simulink model "VTOL_quadplane"  (R2026a)
settings: Solver=ode1  StopTime=120  FixedStep=1/60  MaxStep=0.01
undefined symbols (not defined in the file or in its folder): op_trim, params, Receive, Send
libraries: slpidlib x32, simulink_extras x11, simulink x2, aerolibfltsims x2, aerolibobsolete x1, sim3dlib x1, uavsim3dlib x1
(part 1 of 4)
settings Model: Creator=Admin  LastModifiedBy=Admin
settings DebuggingCC: InheritedTsInSrcMsg=none

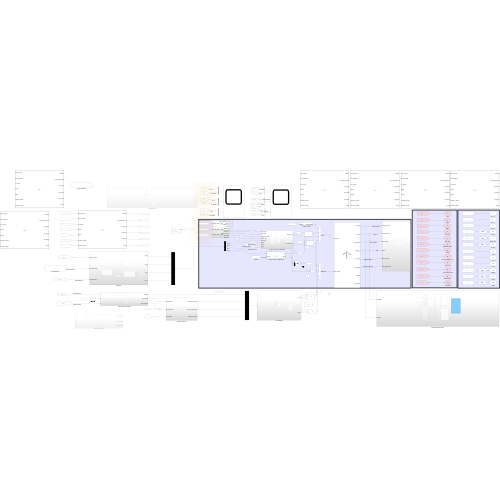
[thumbnail: Simulink's stored preview of the top-level diagram]
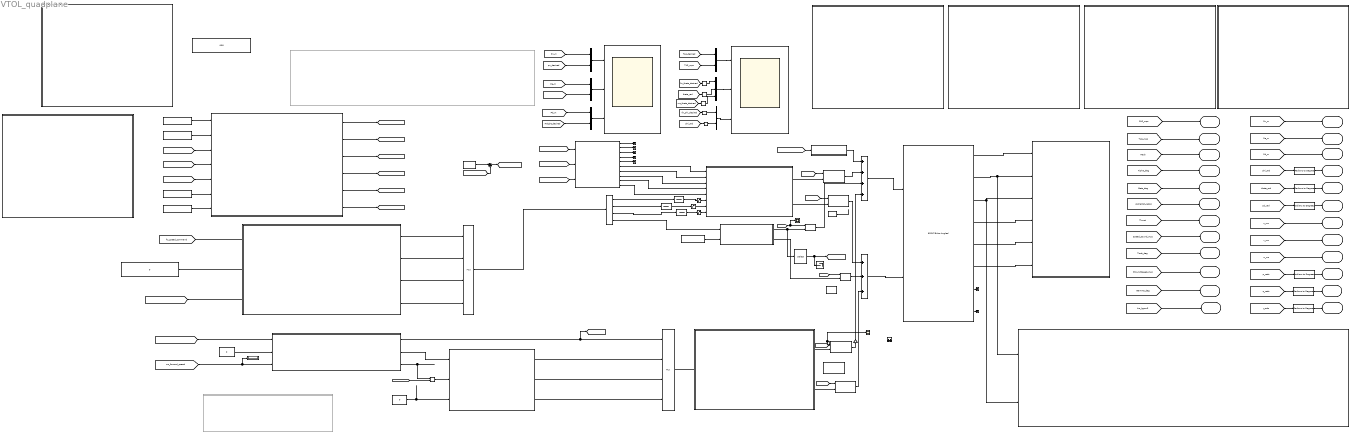
== system VTOL_quadplane ==
  note: Fixed Wing Dynamics
  6DOF (Euler Angles) : aerolibobsolete/6DOF (Euler Angles)  units=Metric (MKS)  mtype=Fixed  rep=Euler Angles  xme_0=[0;0;-1]  Vm_0=[0.01;0;0]  eul_0=[0;0;0]  pm_0=[0;0;0]  mass_0=params.geometric.mass  mass_e=0.5  mass_f=2.0  inertia=params.geometric.I  inertia_e=eye(3)  inertia_f=2*eye(3)  k_quat=1.0  vre_flag=on  abi_flag=off  aMode=0  xme_statename=''  Vm_statename=''  eul_statename=''  quat_statename=''  pm_statename=''  mass_statename=''
  Actuator_servo 1 : TransferFcn  Denominator=[0.02 1]
  Actuator_servo 2 : TransferFcn  Denominator=[0.02 1]
  Actuator_servo 3 : TransferFcn  Denominator=[0.02 1]
  Add : Sum  Inputs=++++
  Add1 : Sum  Inputs=+++
  Add3 : Sum
  Aero_Forces_and_Moments : Subsystem
  Attitude Controller : Subsystem
  Autopilot : Subsystem
  Constant : Constant  Value=24
  Constant1 : Constant  Value=0
  Constant2 : Constant  Value=0
  Constant3 : Constant  Value=-75
  Constant4 : Constant  Value=18
  Constant5 : Constant  Value=0
  Constant7 : Constant
  Constant9 : Constant  Value=-50
  Course Desired : Constant  Value=0
  Course Desired1 : Constant  Value=-100
  Demux : Demux
  Display1 : Display
  Gain : Gain
  Gravity_forces : Subsystem
  MATLAB Function1 : MATLAB Function  TreatAsAtomicUnit=on
  MATLAB Function2 : MATLAB Function  TreatAsAtomicUnit=on
  MATLAB Function3 : MATLAB Function  TreatAsAtomicUnit=on
  MATLAB Function4 : MATLAB Function  TreatAsAtomicUnit=on
  MATLAB Function5 : MATLAB Function  TreatAsAtomicUnit=on
  MATLAB Function6 : MATLAB Function  TreatAsAtomicUnit=on
  MATLAB Function7 : MATLAB Function  TreatAsAtomicUnit=on
  Motor Mixing : Subsystem
  Mux{,1,4,6..7} (5 alike) : Mux  Inputs=2
  Mux2 : Mux
  Mux5 : Mux  Inputs=3
  Mux8 : Mux
  Position Controller1 : Subsystem  Commented=on
  Product{,1..5,8..10} (9 alike) : Product
  Pusher Forces and Moments : MATLAB Function  TreatAsAtomicUnit=on
  Quad Velocity Controller : Subsystem
  Radians to Degrees{,1..4,11..16} (11 alike) : simulink_extras/Transformations/Radians to Degrees
  Saturation1 : Saturate  UpperLimit=deg2rad(25)  LowerLimit=deg2rad(-25)
  Saturation2 : Saturate  UpperLimit=deg2rad(25)  LowerLimit=deg2rad(-25)
  Saturation4 : Saturate  UpperLimit=deg2rad(25)  LowerLimit=deg2rad(-25)
  Scope : Scope  NumInputPorts=3
      settings: ActiveDisplayYMinimum=-441.15296890971007  ActiveDisplayYMaximum=3970.3767201873916
  Scope1 : Scope  NumInputPorts=3
      settings: ActiveDisplayYMinimum=-3.1220021954441637  ActiveDisplayYMaximum=28.098019758997481
  Scope2 : Scope
      settings: ActiveDisplayYMinimum=-1  ActiveDisplayYMaximum=1  DataLoggingVariableName=ScopeData2
  Scope3 : Scope
      settings: ActiveDisplayYMinimum=-0.12499999999999997  ActiveDisplayYMaximum=1.125  DataLoggingVariableName=ScopeData3
  Selector : Selector  InputPortWidth=3  IndexOptions=Index vector (dialog)  Indices=[1]  OutputSizes=1
  Subsystem1 : Subsystem
  Subsystem2 : Subsystem
  Sum : Sum  Inputs=|+-
  Terminator{1..8} (8 alike) : Terminator
  Transition Block : Subsystem  Commented=on
  Visualisation Subsystem : Subsystem
  params1 : Constant  Value=params  OutDataTypeStr=Bus: slBus1
  CAS : Outport
  TAS : Outport  Port=2
  Mach : Outport  Port=3
  Alpha_deg : Outport  Port=4
  Beta_deg : Outport  Port=5
  AlphaDot_radps : Outport  Port=6
  Pn_m : Outport  Port=7
  Pe_m : Outport  Port=8
  Pd_m : Outport  Port=9
  Phi_deg : Outport  Port=10
  Theta_deg : Outport  Port=11
  Psi_deg : Outport  Port=12
  u_ms : Outport  Port=13
  v_ms : Outport  Port=14
  w_ms : Outport  Port=15
  p_deg/s : Outport  Port=16
  q_deg/s : Outport  Port=17
  r_deg/s : Outport  Port=18
  Thrust : Outport  Port=19
  Speed_Sound_mps : Outport  Port=20
  Track_deg : Outport  Port=21
  Ground Speed m/s : Outport  Port=22
  rho_kgpm3 : Outport  Port=23
  Gamma_deg : Outport  Port=24
  tag scope: Thrust=global, fw_height_command=global, fw_speed_command=global, lambda=global, mc_forward_speed=global, mc_height_command=global, mode=global, one_minus_lambda=global, throttle=global
  wires:
  [CAS_mps] -> CAS/1
  [TAS_mps] -> TAS/1
  [Mach] -> Mach/1
  [Alpha_deg] -> Alpha_deg/1
  [Beta_deg] -> Beta_deg/1
  [AlphaDot_radps] -> AlphaDot_radps/1
  [Pn_m] -> Pn_m/1
  [Pe_m] -> Pe_m/1
  [Pd_m] -> Pd_m/1
  [phi_rad] -> Radians to Degrees11/1
  Radians to Degrees11/1 -> Phi_deg/1
  Radians to Degrees12/1 -> Theta_deg/1
  [theta_rad] -> Radians to Degrees12/1
  Radians to Degrees13/1 -> Psi_deg/1
  [psi_rad] -> Radians to Degrees13/1
  [u_ms] -> u_ms/1
  [v_ms] -> v_ms/1
  [w_ms] -> w_ms/1
  [p_rads] -> Radians to Degrees14/1
  Radians to Degrees14/1 -> p_deg/s/1
  [q_rads] -> Radians to Degrees15/1
  Radians to Degrees15/1 -> q_deg/s/1
  [r_rads] -> Radians to Degrees16/1
  Radians to Degrees16/1 -> r_deg/s/1
  [Thrust] -> Thrust/1
  [Speed_Sound_mps] -> Speed_Sound_mps/1
  [Track_deg] -> Track_deg/1
  [GroundSpeed_mps] -> Ground Speed m/s/1
  [rho_kgpm3] -> rho_kgpm3/1
  [Gamma_deg] -> Gamma_deg/1
  ? -> ?
  Course Desired/1 -> Autopilot/2(Course Desired)  "Course Desired"
  Autopilot/1(Del_a) -> Mux8/1
  Autopilot/2(Del_e) -> Mux8/2
  Autopilot/3(Del_r) -> Mux8/3
  Autopilot/4(Del_T) -> Mux8/4
  Subsystem1/5(CAS_mps) -> Terminator5/1
  6DOF (Euler Angles)/3 -> Visualisation Subsystem/2(Rotation), Subsystem2/3(Euler angles)  "Euler angles"
  6DOF (Euler Angles)/1 -> Subsystem2/1(Inertial_Velocity)  "Inertial Velocity"
  [Inertial_Wind_Z] -> Subsystem1/3(Inertial_Wind_Z_mps)
  params1/1 -> Pusher Forces and Moments/2(params)
  Subsystem1/3(Pressure_Pa) -> Terminator3/1
  Subsystem1/4(Mach) -> Terminator4/1
  [Inertial_Wind_X] -> Subsystem1/1(Inertial_Wind_X_mps)
  Aero_Forces_and_Moments/2(Aero_Moments) -> Product3/2
  Subsystem1/9(Alpha_deg) -> Aero_Forces_and_Moments/4(Alpha_deg)
  Add1/1 -> 6DOF (Euler Angles)/2  "Moments"
  Subsystem1/2(Temp k) -> Terminator2/1
  6DOF (Euler Angles)/5 -> Subsystem2/5(Body Velocities)  "Body Velocities"
  6DOF (Euler Angles)/8 -> Terminator7/1
  Demux/1 -> Actuator_servo 1/1  "Del_a"
  Subsystem1/6(rho_kgpm3) -> Aero_Forces_and_Moments/1(rho_kgpm)
  Subsystem1/8(AlphaDot_radps) -> Aero_Forces_and_Moments/3(AlphaDot_radps)
  Subsystem1/1(Speed_Sound_mps) -> Terminator1/1
  6DOF (Euler Angles)/7 -> Terminator6/1
  Subsystem1/7(TAS_mps) -> Aero_Forces_and_Moments/2(TAS_mps)
  Add/1 -> 6DOF (Euler Angles)/1  "forces"
  [DCM] -> Gravity_forces/1(DCM)
  6DOF (Euler Angles)/4 -> Subsystem2/4(DCM)  "DCM"
  Subsystem1/10(Beta_deg) -> Aero_Forces_and_Moments/5(Beta_deg)
  Gravity_forces/1(Gravity_forces) -> Add/1
  [Inertial_Wind_Y] -> Subsystem1/2(Inertial_Wind_Y_mps)
  6DOF (Euler Angles)/2 -> Visualisation Subsystem/1(Translation), Subsystem2/2(Inertial_Position)  "Postion"
  Selector/1 -> [Thrust], Terminator8/1
  6DOF (Euler Angles)/6 -> Subsystem2/6(body angular rates)  "body angular rates"
  Mux8/1 -> Demux/1
  Quad Velocity Controller/1(Throttle) -> [throttle], Mux2/1
  Mux2/1 -> Motor Mixing/1(In1)
  Attitude Controller/1(Roll Control Torque) -> Mux2/2
  Attitude Controller/2(Pitch Control Torque) -> Mux2/3
  [mc_height_command] -> Quad Velocity Controller/1(In1)  "Height Desired"
  Attitude Controller/3(Yaw Control Torque) -> Mux2/4
  Constant2/1 -> Quad Velocity Controller/2(In2)
  Motor Mixing/1(F_vtol) -> Product1/2
  Motor Mixing/2(M_xyz) -> Product/2
  Constant5/1 -> Attitude Controller/3(Psi_desired)
  Product/1 -> Add1/3
  [Pd_m] -> Mux7/1  "Pd_m"
  [Pn_m] -> Mux1/1  "Pn_m"
  [pe_desired] -> Mux/2  "pe_desired"
  [Pe_m] -> Mux/1  "pe_m"
  Mux1/1 -> Scope/1
  [pn_desired] -> Mux1/2  "pn_desired"
  [Height_desired] -> Mux7/2  "Pd_desired"
  Mux/1 -> Scope/2
  Mux7/1 -> Scope/3
  [one_minus_lambda] -> Product/1
  [one_minus_lambda] -> Scope2/1, Product1/1
  Product1/1 -> Gain/1
  Aero_Forces_and_Moments/1(Aero_forces) -> Product2/2
  [lambda] -> Product2/1
  Product3/1 -> Add1/1
  [lambda] -> Product3/1
  Product2/1 -> Add/2
  Mux4/1 -> Scope1/1
  Mux5/1 -> Scope1/2
  Mux6/1 -> Scope1/3
  [Tas_desired] -> Mux4/1  "V-desired"
  [TAS_mps] -> Mux4/2  "Vms"
  [fw_theta_desired] -> Radians to Degrees/1
  [theta_rad] -> Radians to Degrees1/1
  [fw_phi_desired] -> Radians to Degrees2/1
  Radians to Degrees/1 -> Mux5/1  "Theta_desired"
  Radians to Degrees1/1 -> Mux5/2  "Theta"
  Radians to Degrees2/1 -> Mux6/1  "Phi_desired"
  [phi_rad] -> Radians to Degrees3/1
  Radians to Degrees3/1 -> Mux6/2  "Phi"
  Quad Velocity Controller/2(Phi_desired) -> Attitude Controller/1(Phi_desired)
  [fw_height_command] -> Autopilot/3(Height Desired)  "Height Desired"
  Constant1/1 -> ?
  Constant7/1 -> Sum/1
  Demux/4 -> Pusher Forces and Moments/1(u)  "Del_T"
  [lambda] -> Sum/2
  Sum/1 -> [one_minus_lambda]
  Actuator_servo 1/1 -> Saturation4/1
  Actuator_servo 2/1 -> Saturation1/1
  Actuator_servo 3/1 -> Saturation2/1
  [mc_forward_speed] -> Display1/1, Quad Velocity Controller/3(In3)  "Height Desired"
  [lambda] -> Product9/1, Scope3/1
  Pusher Forces and Moments/2(M_fw) -> Product5/2
  [lambda] -> Product5/1
  Quad Velocity Controller/3(Theta_desired) -> Product8/1
  Demux/3 -> Actuator_servo 3/1  "Del_r"
  Demux/2 -> Actuator_servo 2/1  "Del_e"
  [fw_speed_command] -> Autopilot/1(Speed_desired)  "Speed_desired"
  Pusher Forces and Moments/1(F_fw) -> Product9/2, Selector/1
  Product5/1 -> Add1/2
  Saturation4/1 -> Aero_Forces_and_Moments/6(Del_a)
  Saturation2/1 -> Aero_Forces_and_Moments/8(Del_r)
  Constant/1 -> MATLAB Function1/1(cruise_speed)
  MATLAB Function1/5(fw_height) -> [fw_height_command]
  Constant4/1 -> MATLAB Function1/6(transition_speed)
  MATLAB Function1/2(mc_forward_speed) -> [mc_forward_speed]
  Constant3/1 -> MATLAB Function1/2(cruise_altitude)
  MATLAB Function1/3(mc_height) -> [mc_height_command]
  MATLAB Function1/4(fw_speed) -> [fw_speed_command]
  [Pd_m] -> MATLAB Function1/5(height)
  Constant9/1 -> MATLAB Function1/7(transition_height)
  MATLAB Function1/6(mode) -> [mode]
  MATLAB Function1/1(lambda) -> [lambda]
  [TAS_mps] -> MATLAB Function1/3(mc_speed)
  [TAS_mps] -> MATLAB Function1/4(speed)
  [one_minus_lambda] -> Product8/2
  Product8/1 -> Attitude Controller/2(Theta_desired)
  Product9/1 -> Add/3
  Gain/1 -> Add/4
  Saturation1/1 -> Aero_Forces_and_Moments/7(Del_e)
  [mc_theta_desired] -> Radians to Degrees4/1
  Radians to Degrees4/1 -> Mux5/3  "mc_Theta_desired"

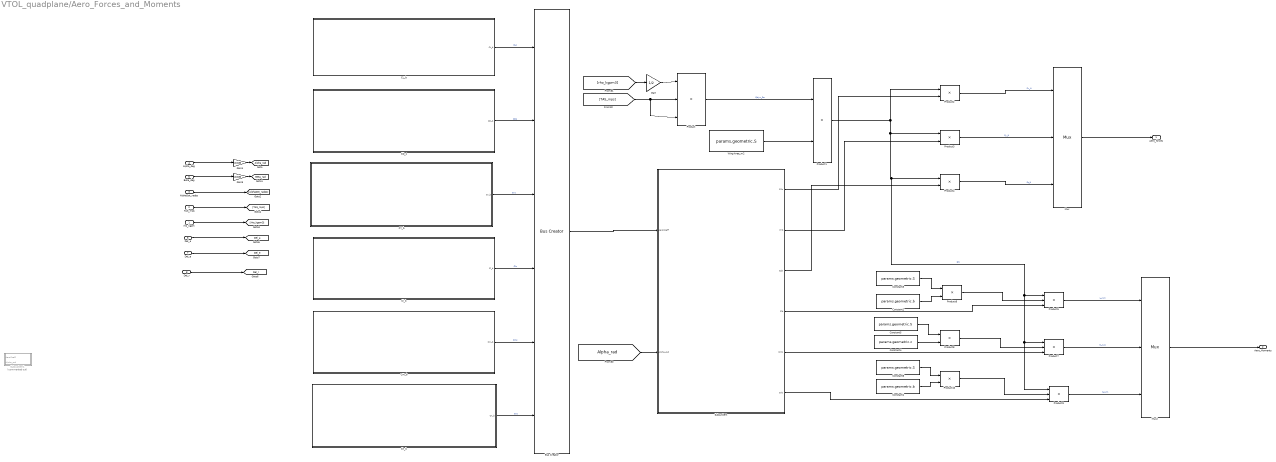
== system VTOL_quadplane/Aero_Forces_and_Moments ==
  rho_kgpm : Inport
  TAS_mps : Inport  Port=2
  AlphaDot_radps : Inport  Port=3
  Alpha_deg : Inport  Port=4
  Beta_deg : Inport  Port=5
  Del_a : Inport  Port=6
  Del_e : Inport  Port=7
  Del_r : Inport  Port=8
  Bus Creator : BusCreator  Inputs=6
  CD_s : Subsystem
  CL_b : Subsystem
  CY_b : Subsystem
  Cl_b : Subsystem
  Cm_b : Subsystem
  Cn_b : Subsystem
  Constant1 : Constant  Value=params.geometric.b
  Constant2 : Constant  Value=params.geometric.b
  Constant3 : Constant  Value=params.geometric.S
  Constant4 : Constant  Value=params.geometric.c
  Constant5 : Constant  Value=params.geometric.S
  Constant6 : Constant  Value=params.geometric.S
  Gain : Gain  Gain=1/2
  Gain4 : Gain  Gain=pi/180
  Gain5 : Gain  Gain=pi/180
  Mux : Mux  Inputs=3
  Mux2 : Mux  Inputs=3
  Product{,5,7,9} (4 alike) : Product  Inputs=3
  Product{1..4,6,8,10} (7 alike) : Product
  Subsystem : Subsystem
  Subsystem1 : Subsystem  Commented=on
  Wing Area_m2 : Constant  Value=params.geometric.S
  Aero_forces : Outport
  Aero_Moments : Outport  Port=2
  tag scope: Alpha_rad=global, Beta_rad=global, Del_a=global, Del_e=global, Del_r=global
  wires:
  Subsystem/5(Cmb) -> Product7/3
  Product5/1 -> Mux2/1  "L_n/m"
  Wing Area_m2/1 -> Product1/2
  CD_s/1(CD_b) -> Bus Creator/2  "CDs"
  [TAS_mps] -> Product/3, Product/2
  Product/1 -> Product1/1  "Qdyn_Pa"
  Product1/1 -> Product9/1, Product7/1, Product5/1, Product4/1, Product3/1, Product2/1  "QS"
  Bus Creator/1 -> Subsystem/1(AeroCoeff)
  Constant6/1 -> Product10/1
  Product7/1 -> Mux2/2  "M_n/m"
  Mux2/1 -> Aero_Moments/1
  [Alpha_rad] -> Subsystem/2(Alpha_rad)
  [rho_kgpm3] -> Gain/1
  CY_b/1(CY_b) -> Bus Creator/3  "CYs"
  Product10/1 -> Product9/2
  Gain/1 -> Product/1
  Product9/1 -> Mux2/3  "N_n/m"
  Subsystem/4(Clb) -> Product5/3
  Product8/1 -> Product7/2
  Cm_b/1(Cm_b) -> Bus Creator/5  "Cms"
  Product2/1 -> Mux/1  "Fx_N"
  Product3/1 -> Mux/2  "Fy_N"
  Constant5/1 -> Product8/1
  Constant2/1 -> Product6/2
  Product6/1 -> Product5/2
  Constant3/1 -> Product6/1
  AlphaDot_radps/1 -> [AlphaDot_radps]
  Subsystem/1(CXb) -> Product2/2
  Alpha_deg/1 -> Gain4/1
  Constant4/1 -> Product8/2
  Subsystem/2(CYb) -> Product3/2
  Product4/1 -> Mux/3  "Fz_N"
  Beta_deg/1 -> Gain5/1
  CL_b/1(CL_b) -> Bus Creator/1  "CLs"
  TAS_mps/1 -> [TAS_mps]
  Cl_b/1(Cl_b) -> Bus Creator/4  "Cls"
  Subsystem/6(Cnb) -> Product9/3
  Del_r/1 -> [Del_r]
  Gain4/1 -> [Alpha_rad]
  Gain5/1 -> [Beta_rad]
  Constant1/1 -> Product10/2
  Del_e/1 -> [Del_e]
  Subsystem/3(CZb) -> Product4/2
  Cn_b/1(Cn_b) -> Bus Creator/6  "Cns"
  Mux/1 -> Aero_forces/1
  Del_a/1 -> [Del_a]
  rho_kgpm/1 -> [rho_kgpm3]

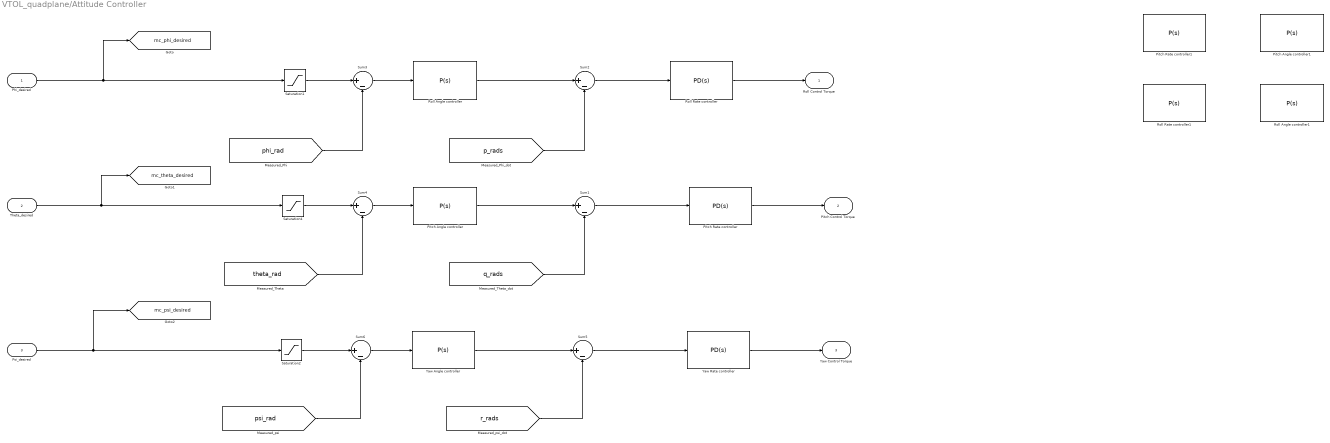
== system VTOL_quadplane/Attitude Controller ==
  Phi_desired : Inport
  Theta_desired : Inport  Port=2
  Psi_desired : Inport  Port=3
  Pitch Angle controller : slpidlib/PID Controller  Controller=P  Form=Parallel  TimeDomain=Continuous-time  UseExternalTs=off  SampleTime=-1  IntegratorMethod=Forward Euler  FilterMethod=Forward Euler  ControllerParametersSource=internal  P=4.9  I=8.92  UseKiTs=off  D=0.101  UseExternalDerivativeSource=off  N=50  UseFilter=on  TunerSelectOption=Transfer Function Based (PID Tuner App)  InitialConditionSource=internal  InitialConditionForIntegrator=0  InitialConditionForFilter=0  DifferentiatorICPrevScaledInput=0  ExternalReset=none  TrackingMode=off  Kt=1  LimitOutput=off  SatLimitsSource=internal  UpperSaturationLimit=inf  LowerSaturationLimit=-inf  LinearizeAsGain=on  AntiWindupMode=none  Kb=1  LimitIntegrator=off  UpperIntegratorSaturationLimit=inf  LowerIntegratorSaturationLimit=-inf  POutMin=[]  POutMax=[]  IOutMin=[]  IOutMax=[]  DOutMin=[]  DOutMax=[]  NOutMin=[]  NOutMax=[]  SumOutMin=[]  SumOutMax=[]  SaturationOutMin=[]  SaturationOutMax=[]  PParamMin=[]  PParamMax=[]  IParamMin=[]  IParamMax=[]  DParamMin=[]  DParamMax=[]  NParamMin=[]  NParamMax=[]  KbParamMin=[]  KbParamMax=[]  KtParamMin=[]  KtParamMax=[]  KbOutMin=[]  KbOutMax=[]  KtOutMin=[]  KtOutMax=[]  IntegratorOutMin=[]  IntegratorOutMax=[]  FilterOutMin=[]  FilterOutMax=[]  SumI1OutMin=[]  SumI1OutMax=[]  SumI2OutMin=[]  SumI2OutMax=[]  SumI3OutMin=[]  SumI3OutMax=[]  SumI4OutMin=[]  SumI4OutMax=[]  SumDOutMin=[]  SumDOutMax=[]  DifferentiatorOutMin=[]  DifferentiatorOutMax=[]  FilterDiffOutCoefMin=[]  FilterDiffOutCoefMax=[]  ReciprocalOutMin=[]  ReciprocalOutMax=[]  SumDenOutMin=[]  SumDenOutMax=[]  SumNumOutMin=[]  SumNumOutMax=[]  DivideOutMin=[]  DivideOutMax=[]  UdiffTsProdOutMin=[]  UdiffTsProdOutMax=[]  NTsProdOutMin=[]  NTsProdOutMax=[]  UintegralTsProdOutMin=[]  UintegralTsProdOutMax=[]  UngainTsProdOutMin=[]  UngainTsProdOutMax=[]  ClampingZeroOutDataTypeStr=Inherit: Inherit via back propagation  ClampingZeroOutMin=[]  ClampingZeroOutMax=[]  FilterDenConstantOutDataTypeStr=Inherit: Inherit via back propagation  FilterDenConstantOutMin=[]  FilterDenConstantOutMax=[]  PCopyOutDataTypeStr=Inherit: Inherit via back propagation  PCopyOutMin=[]  PCopyOutMax=[]  NCopyOutDataTypeStr=Inherit: Inherit via back propagation  NCopyOutMin=[]  NCopyOutMax=[]  IntegratorContinuousStateAttributes=''  IntegratorStateMustResolveToSignalObject=off  IntegratorRTWStateStorageClass=Auto  FilterContinuousStateAttributes=''  FilterStateMustResolveToSignalObject=off  FilterRTWStateStorageClass=Auto  ParallelPVariant=InternalParameters  IdealPVariant=Disabled  IVariant=Disabled  DVariant=Disabled  IntegratorVariant=Disabled  SatVariant=Disabled  AWVariant=Disabled  PCopyVariant=Disabled  TRVariant=Disabled  FdbkBlocksVariant=Forward  IdealPFdbkVariant=Disabled  SatFdbkVariant=Disabled  DerivativeFilterVariant=Disabled  NVariant=Disabled  NCopyVariant=Disabled_SignalSpec  FilterICVariant=Disabled  IntegratorICVariant=Disabled  ExternalResetVariant=Disabled  TRSumVariant=Passthrough  SumFdbkVariant=Disabled  SumVariant=Passthrough_P  TsampFilterVariant=InternalTs  TsampNgainVariant=Passthrough  TsampIntegralVariant=Disabled_SignalSpec  ExternalSaturationOutDataTypeStr=Inherit: Same as second input  DerivativeSourceVariant=Disabled  PreIntVariant=InternalPreInt
  Pitch Angle controller1 : slpidlib/PID Controller  Controller=P  Form=Parallel  TimeDomain=Continuous-time  UseExternalTs=off  SampleTime=-1  IntegratorMethod=Forward Euler  FilterMethod=Forward Euler  ControllerParametersSource=internal  P=2.07  I=8.92  UseKiTs=off  D=0.101  UseExternalDerivativeSource=off  N=50  UseFilter=on  TunerSelectOption=Transfer Function Based (PID Tuner App)  InitialConditionSource=internal  InitialConditionForIntegrator=0  InitialConditionForFilter=0  DifferentiatorICPrevScaledInput=0  ExternalReset=none  TrackingMode=off  Kt=1  LimitOutput=off  SatLimitsSource=internal  UpperSaturationLimit=inf  LowerSaturationLimit=-inf  LinearizeAsGain=on  AntiWindupMode=none  Kb=1  LimitIntegrator=off  UpperIntegratorSaturationLimit=inf  LowerIntegratorSaturationLimit=-inf  POutMin=[]  POutMax=[]  IOutMin=[]  IOutMax=[]  DOutMin=[]  DOutMax=[]  NOutMin=[]  NOutMax=[]  SumOutMin=[]  SumOutMax=[]  SaturationOutMin=[]  SaturationOutMax=[]  PParamMin=[]  PParamMax=[]  IParamMin=[]  IParamMax=[]  DParamMin=[]  DParamMax=[]  NParamMin=[]  NParamMax=[]  KbParamMin=[]  KbParamMax=[]  KtParamMin=[]  KtParamMax=[]  KbOutMin=[]  KbOutMax=[]  KtOutMin=[]  KtOutMax=[]  IntegratorOutMin=[]  IntegratorOutMax=[]  FilterOutMin=[]  FilterOutMax=[]  SumI1OutMin=[]  SumI1OutMax=[]  SumI2OutMin=[]  SumI2OutMax=[]  SumI3OutMin=[]  SumI3OutMax=[]  SumI4OutMin=[]  SumI4OutMax=[]  SumDOutMin=[]  SumDOutMax=[]  DifferentiatorOutMin=[]  DifferentiatorOutMax=[]  FilterDiffOutCoefMin=[]  FilterDiffOutCoefMax=[]  ReciprocalOutMin=[]  ReciprocalOutMax=[]  SumDenOutMin=[]  SumDenOutMax=[]  SumNumOutMin=[]  SumNumOutMax=[]  DivideOutMin=[]  DivideOutMax=[]  UdiffTsProdOutMin=[]  UdiffTsProdOutMax=[]  NTsProdOutMin=[]  NTsProdOutMax=[]  UintegralTsProdOutMin=[]  UintegralTsProdOutMax=[]  UngainTsProdOutMin=[]  UngainTsProdOutMax=[]  ClampingZeroOutDataTypeStr=Inherit: Inherit via back propagation  ClampingZeroOutMin=[]  ClampingZeroOutMax=[]  FilterDenConstantOutDataTypeStr=Inherit: Inherit via back propagation  FilterDenConstantOutMin=[]  FilterDenConstantOutMax=[]  PCopyOutDataTypeStr=Inherit: Inherit via back propagation  PCopyOutMin=[]  PCopyOutMax=[]  NCopyOutDataTypeStr=Inherit: Inherit via back propagation  NCopyOutMin=[]  NCopyOutMax=[]  IntegratorContinuousStateAttributes=''  IntegratorStateMustResolveToSignalObject=off  IntegratorRTWStateStorageClass=Auto  FilterContinuousStateAttributes=''  FilterStateMustResolveToSignalObject=off  FilterRTWStateStorageClass=Auto  ParallelPVariant=InternalParameters  IdealPVariant=Disabled  IVariant=Disabled  DVariant=Disabled  IntegratorVariant=Disabled  SatVariant=Disabled  AWVariant=Disabled  PCopyVariant=Disabled  TRVariant=Disabled  FdbkBlocksVariant=Forward  IdealPFdbkVariant=Disabled  SatFdbkVariant=Disabled  DerivativeFilterVariant=Disabled  NVariant=Disabled  NCopyVariant=Disabled_SignalSpec  FilterICVariant=Disabled  IntegratorICVariant=Disabled  ExternalResetVariant=Disabled  TRSumVariant=Passthrough  SumFdbkVariant=Disabled  SumVariant=Passthrough_P  TsampFilterVariant=InternalTs  TsampNgainVariant=Passthrough  TsampIntegralVariant=Disabled_SignalSpec  ExternalSaturationOutDataTypeStr=Inherit: Same as second input  DerivativeSourceVariant=Disabled  PreIntVariant=InternalPreInt
  Pitch Rate controller : slpidlib/PID Controller  Controller=PD  Form=Parallel  TimeDomain=Continuous-time  UseExternalTs=off  SampleTime=-1  IntegratorMethod=Forward Euler  FilterMethod=Forward Euler  ControllerParametersSource=internal  P=0.154  I=8.92  UseKiTs=off  D=0.000216  UseExternalDerivativeSource=off  N=100  UseFilter=on  TunerSelectOption=Transfer Function Based (PID Tuner App)  InitialConditionSource=internal  InitialConditionForIntegrator=0  InitialConditionForFilter=0  DifferentiatorICPrevScaledInput=0  ExternalReset=none  TrackingMode=off  Kt=1  LimitOutput=off  SatLimitsSource=internal  UpperSaturationLimit=inf  LowerSaturationLimit=-inf  LinearizeAsGain=on  AntiWindupMode=none  Kb=1  LimitIntegrator=off  UpperIntegratorSaturationLimit=inf  LowerIntegratorSaturationLimit=-inf  POutMin=[]  POutMax=[]  IOutMin=[]  IOutMax=[]  DOutMin=[]  DOutMax=[]  NOutMin=[]  NOutMax=[]  SumOutMin=[]  SumOutMax=[]  SaturationOutMin=[]  SaturationOutMax=[]  PParamMin=[]  PParamMax=[]  IParamMin=[]  IParamMax=[]  DParamMin=[]  DParamMax=[]  NParamMin=[]  NParamMax=[]  KbParamMin=[]  KbParamMax=[]  KtParamMin=[]  KtParamMax=[]  KbOutMin=[]  KbOutMax=[]  KtOutMin=[]  KtOutMax=[]  IntegratorOutMin=[]  IntegratorOutMax=[]  FilterOutMin=[]  FilterOutMax=[]  SumI1OutMin=[]  SumI1OutMax=[]  SumI2OutMin=[]  SumI2OutMax=[]  SumI3OutMin=[]  SumI3OutMax=[]  SumI4OutMin=[]  SumI4OutMax=[]  SumDOutMin=[]  SumDOutMax=[]  DifferentiatorOutMin=[]  DifferentiatorOutMax=[]  FilterDiffOutCoefMin=[]  FilterDiffOutCoefMax=[]  ReciprocalOutMin=[]  ReciprocalOutMax=[]  SumDenOutMin=[]  SumDenOutMax=[]  SumNumOutMin=[]  SumNumOutMax=[]  DivideOutMin=[]  DivideOutMax=[]  UdiffTsProdOutMin=[]  UdiffTsProdOutMax=[]  NTsProdOutMin=[]  NTsProdOutMax=[]  UintegralTsProdOutMin=[]  UintegralTsProdOutMax=[]  UngainTsProdOutMin=[]  UngainTsProdOutMax=[]  ClampingZeroOutDataTypeStr=Inherit: Inherit via back propagation  ClampingZeroOutMin=[]  ClampingZeroOutMax=[]  FilterDenConstantOutDataTypeStr=Inherit: Inherit via back propagation  FilterDenConstantOutMin=[]  FilterDenConstantOutMax=[]  PCopyOutDataTypeStr=Inherit: Inherit via back propagation  PCopyOutMin=[]  PCopyOutMax=[]  NCopyOutDataTypeStr=Inherit: Inherit via back propagation  NCopyOutMin=[]  NCopyOutMax=[]  IntegratorContinuousStateAttributes=''  IntegratorStateMustResolveToSignalObject=off  IntegratorRTWStateStorageClass=Auto  FilterContinuousStateAttributes=''  FilterStateMustResolveToSignalObject=off  FilterRTWStateStorageClass=Auto  ParallelPVariant=InternalParameters  IdealPVariant=Disabled  IVariant=Disabled  DVariant=InternalParameters  IntegratorVariant=Disabled  SatVariant=Disabled  AWVariant=Disabled  PCopyVariant=Disabled  TRVariant=Disabled  FdbkBlocksVariant=Forward  IdealPFdbkVariant=Disabled  SatFdbkVariant=Disabled  DerivativeFilterVariant=ContFilter  NVariant=InternalParameters  NCopyVariant=Disabled  FilterICVariant=InternalICsFilter  IntegratorICVariant=Disabled  ExternalResetVariant=Disabled  TRSumVariant=Passthrough  SumFdbkVariant=Disabled  SumVariant=Sum_PD  TsampFilterVariant=InternalTs  TsampNgainVariant=Passthrough  TsampIntegralVariant=Disabled_SignalSpec  ExternalSaturationOutDataTypeStr=Inherit: Same as second input  DerivativeSourceVariant=ErrorSignal  PreIntVariant=InternalPreInt
  Pitch Rate controller1 : slpidlib/PID Controller  Controller=P  Form=Parallel  TimeDomain=Continuous-time  UseExternalTs=off  SampleTime=-1  IntegratorMethod=Forward Euler  FilterMethod=Forward Euler  ControllerParametersSource=internal  P=0.0818  I=8.92  UseKiTs=off  D=0.0115  UseExternalDerivativeSource=off  N=50  UseFilter=on  TunerSelectOption=Transfer Function Based (PID Tuner App)  InitialConditionSource=internal  InitialConditionForIntegrator=0  InitialConditionForFilter=0  DifferentiatorICPrevScaledInput=0  ExternalReset=none  TrackingMode=off  Kt=1  LimitOutput=off  SatLimitsSource=internal  UpperSaturationLimit=inf  LowerSaturationLimit=-inf  LinearizeAsGain=on  AntiWindupMode=none  Kb=1  LimitIntegrator=off  UpperIntegratorSaturationLimit=inf  LowerIntegratorSaturationLimit=-inf  POutMin=[]  POutMax=[]  IOutMin=[]  IOutMax=[]  DOutMin=[]  DOutMax=[]  NOutMin=[]  NOutMax=[]  SumOutMin=[]  SumOutMax=[]  SaturationOutMin=[]  SaturationOutMax=[]  PParamMin=[]  PParamMax=[]  IParamMin=[]  IParamMax=[]  DParamMin=[]  DParamMax=[]  NParamMin=[]  NParamMax=[]  KbParamMin=[]  KbParamMax=[]  KtParamMin=[]  KtParamMax=[]  KbOutMin=[]  KbOutMax=[]  KtOutMin=[]  KtOutMax=[]  IntegratorOutMin=[]  IntegratorOutMax=[]  FilterOutMin=[]  FilterOutMax=[]  SumI1OutMin=[]  SumI1OutMax=[]  SumI2OutMin=[]  SumI2OutMax=[]  SumI3OutMin=[]  SumI3OutMax=[]  SumI4OutMin=[]  SumI4OutMax=[]  SumDOutMin=[]  SumDOutMax=[]  DifferentiatorOutMin=[]  DifferentiatorOutMax=[]  FilterDiffOutCoefMin=[]  FilterDiffOutCoefMax=[]  ReciprocalOutMin=[]  ReciprocalOutMax=[]  SumDenOutMin=[]  SumDenOutMax=[]  SumNumOutMin=[]  SumNumOutMax=[]  DivideOutMin=[]  DivideOutMax=[]  UdiffTsProdOutMin=[]  UdiffTsProdOutMax=[]  NTsProdOutMin=[]  NTsProdOutMax=[]  UintegralTsProdOutMin=[]  UintegralTsProdOutMax=[]  UngainTsProdOutMin=[]  UngainTsProdOutMax=[]  ClampingZeroOutDataTypeStr=Inherit: Inherit via back propagation  ClampingZeroOutMin=[]  ClampingZeroOutMax=[]  FilterDenConstantOutDataTypeStr=Inherit: Inherit via back propagation  FilterDenConstantOutMin=[]  FilterDenConstantOutMax=[]  PCopyOutDataTypeStr=Inherit: Inherit via back propagation  PCopyOutMin=[]  PCopyOutMax=[]  NCopyOutDataTypeStr=Inherit: Inherit via back propagation  NCopyOutMin=[]  NCopyOutMax=[]  IntegratorContinuousStateAttributes=''  IntegratorStateMustResolveToSignalObject=off  IntegratorRTWStateStorageClass=Auto  FilterContinuousStateAttributes=''  FilterStateMustResolveToSignalObject=off  FilterRTWStateStorageClass=Auto  ParallelPVariant=InternalParameters  IdealPVariant=Disabled  IVariant=Disabled  DVariant=Disabled  IntegratorVariant=Disabled  SatVariant=Disabled  AWVariant=Disabled  PCopyVariant=Disabled  TRVariant=Disabled  FdbkBlocksVariant=Forward  IdealPFdbkVariant=Disabled  SatFdbkVariant=Disabled  DerivativeFilterVariant=Disabled  NVariant=Disabled  NCopyVariant=Disabled_SignalSpec  FilterICVariant=Disabled  IntegratorICVariant=Disabled  ExternalResetVariant=Disabled  TRSumVariant=Passthrough  SumFdbkVariant=Disabled  SumVariant=Passthrough_P  TsampFilterVariant=InternalTs  TsampNgainVariant=Passthrough  TsampIntegralVariant=Disabled_SignalSpec  ExternalSaturationOutDataTypeStr=Inherit: Same as second input  DerivativeSourceVariant=Disabled  PreIntVariant=InternalPreInt
  Roll Angle controller : slpidlib/PID Controller  Controller=P  Form=Parallel  TimeDomain=Continuous-time  UseExternalTs=off  SampleTime=-1  IntegratorMethod=Forward Euler  FilterMethod=Forward Euler  ControllerParametersSource=internal  P=4.9  I=8.92  UseKiTs=off  D=0.101  UseExternalDerivativeSource=off  N=50  UseFilter=on  TunerSelectOption=Transfer Function Based (PID Tuner App)  InitialConditionSource=internal  InitialConditionForIntegrator=0  InitialConditionForFilter=0  DifferentiatorICPrevScaledInput=0  ExternalReset=none  TrackingMode=off  Kt=1  LimitOutput=off  SatLimitsSource=internal  UpperSaturationLimit=inf  LowerSaturationLimit=-inf  LinearizeAsGain=on  AntiWindupMode=none  Kb=1  LimitIntegrator=off  UpperIntegratorSaturationLimit=inf  LowerIntegratorSaturationLimit=-inf  POutMin=[]  POutMax=[]  IOutMin=[]  IOutMax=[]  DOutMin=[]  DOutMax=[]  NOutMin=[]  NOutMax=[]  SumOutMin=[]  SumOutMax=[]  SaturationOutMin=[]  SaturationOutMax=[]  PParamMin=[]  PParamMax=[]  IParamMin=[]  IParamMax=[]  DParamMin=[]  DParamMax=[]  NParamMin=[]  NParamMax=[]  KbParamMin=[]  KbParamMax=[]  KtParamMin=[]  KtParamMax=[]  KbOutMin=[]  KbOutMax=[]  KtOutMin=[]  KtOutMax=[]  IntegratorOutMin=[]  IntegratorOutMax=[]  FilterOutMin=[]  FilterOutMax=[]  SumI1OutMin=[]  SumI1OutMax=[]  SumI2OutMin=[]  SumI2OutMax=[]  SumI3OutMin=[]  SumI3OutMax=[]  SumI4OutMin=[]  SumI4OutMax=[]  SumDOutMin=[]  SumDOutMax=[]  DifferentiatorOutMin=[]  DifferentiatorOutMax=[]  FilterDiffOutCoefMin=[]  FilterDiffOutCoefMax=[]  ReciprocalOutMin=[]  ReciprocalOutMax=[]  SumDenOutMin=[]  SumDenOutMax=[]  SumNumOutMin=[]  SumNumOutMax=[]  DivideOutMin=[]  DivideOutMax=[]  UdiffTsProdOutMin=[]  UdiffTsProdOutMax=[]  NTsProdOutMin=[]  NTsProdOutMax=[]  UintegralTsProdOutMin=[]  UintegralTsProdOutMax=[]  UngainTsProdOutMin=[]  UngainTsProdOutMax=[]  ClampingZeroOutDataTypeStr=Inherit: Inherit via back propagation  ClampingZeroOutMin=[]  ClampingZeroOutMax=[]  FilterDenConstantOutDataTypeStr=Inherit: Inherit via back propagation  FilterDenConstantOutMin=[]  FilterDenConstantOutMax=[]  PCopyOutDataTypeStr=Inherit: Inherit via back propagation  PCopyOutMin=[]  PCopyOutMax=[]  NCopyOutDataTypeStr=Inherit: Inherit via back propagation  NCopyOutMin=[]  NCopyOutMax=[]  IntegratorContinuousStateAttributes=''  IntegratorStateMustResolveToSignalObject=off  IntegratorRTWStateStorageClass=Auto  FilterContinuousStateAttributes=''  FilterStateMustResolveToSignalObject=off  FilterRTWStateStorageClass=Auto  ParallelPVariant=InternalParameters  IdealPVariant=Disabled  IVariant=Disabled  DVariant=Disabled  IntegratorVariant=Disabled  SatVariant=Disabled  AWVariant=Disabled  PCopyVariant=Disabled  TRVariant=Disabled  FdbkBlocksVariant=Forward  IdealPFdbkVariant=Disabled  SatFdbkVariant=Disabled  DerivativeFilterVariant=Disabled  NVariant=Disabled  NCopyVariant=Disabled_SignalSpec  FilterICVariant=Disabled  IntegratorICVariant=Disabled  ExternalResetVariant=Disabled  TRSumVariant=Passthrough  SumFdbkVariant=Disabled  SumVariant=Passthrough_P  TsampFilterVariant=InternalTs  TsampNgainVariant=Passthrough  TsampIntegralVariant=Disabled_SignalSpec  ExternalSaturationOutDataTypeStr=Inherit: Same as second input  DerivativeSourceVariant=Disabled  PreIntVariant=InternalPreInt
  Roll Angle controller1 : slpidlib/PID Controller  Controller=P  Form=Parallel  TimeDomain=Continuous-time  UseExternalTs=off  SampleTime=-1  IntegratorMethod=Forward Euler  FilterMethod=Forward Euler  ControllerParametersSource=internal  P=2.07  I=8.92  UseKiTs=off  D=0.101  UseExternalDerivativeSource=off  N=50  UseFilter=on  TunerSelectOption=Transfer Function Based (PID Tuner App)  InitialConditionSource=internal  InitialConditionForIntegrator=0  InitialConditionForFilter=0  DifferentiatorICPrevScaledInput=0  ExternalReset=none  TrackingMode=off  Kt=1  LimitOutput=off  SatLimitsSource=internal  UpperSaturationLimit=inf  LowerSaturationLimit=-inf  LinearizeAsGain=on  AntiWindupMode=none  Kb=1  LimitIntegrator=off  UpperIntegratorSaturationLimit=inf  LowerIntegratorSaturationLimit=-inf  POutMin=[]  POutMax=[]  IOutMin=[]  IOutMax=[]  DOutMin=[]  DOutMax=[]  NOutMin=[]  NOutMax=[]  SumOutMin=[]  SumOutMax=[]  SaturationOutMin=[]  SaturationOutMax=[]  PParamMin=[]  PParamMax=[]  IParamMin=[]  IParamMax=[]  DParamMin=[]  DParamMax=[]  NParamMin=[]  NParamMax=[]  KbParamMin=[]  KbParamMax=[]  KtParamMin=[]  KtParamMax=[]  KbOutMin=[]  KbOutMax=[]  KtOutMin=[]  KtOutMax=[]  IntegratorOutMin=[]  IntegratorOutMax=[]  FilterOutMin=[]  FilterOutMax=[]  SumI1OutMin=[]  SumI1OutMax=[]  SumI2OutMin=[]  SumI2OutMax=[]  SumI3OutMin=[]  SumI3OutMax=[]  SumI4OutMin=[]  SumI4OutMax=[]  SumDOutMin=[]  SumDOutMax=[]  DifferentiatorOutMin=[]  DifferentiatorOutMax=[]  FilterDiffOutCoefMin=[]  FilterDiffOutCoefMax=[]  ReciprocalOutMin=[]  ReciprocalOutMax=[]  SumDenOutMin=[]  SumDenOutMax=[]  SumNumOutMin=[]  SumNumOutMax=[]  DivideOutMin=[]  DivideOutMax=[]  UdiffTsProdOutMin=[]  UdiffTsProdOutMax=[]  NTsProdOutMin=[]  NTsProdOutMax=[]  UintegralTsProdOutMin=[]  UintegralTsProdOutMax=[]  UngainTsProdOutMin=[]  UngainTsProdOutMax=[]  ClampingZeroOutDataTypeStr=Inherit: Inherit via back propagation  ClampingZeroOutMin=[]  ClampingZeroOutMax=[]  FilterDenConstantOutDataTypeStr=Inherit: Inherit via back propagation  FilterDenConstantOutMin=[]  FilterDenConstantOutMax=[]  PCopyOutDataTypeStr=Inherit: Inherit via back propagation  PCopyOutMin=[]  PCopyOutMax=[]  NCopyOutDataTypeStr=Inherit: Inherit via back propagation  NCopyOutMin=[]  NCopyOutMax=[]  IntegratorContinuousStateAttributes=''  IntegratorStateMustResolveToSignalObject=off  IntegratorRTWStateStorageClass=Auto  FilterContinuousStateAttributes=''  FilterStateMustResolveToSignalObject=off  FilterRTWStateStorageClass=Auto  ParallelPVariant=InternalParameters  IdealPVariant=Disabled  IVariant=Disabled  DVariant=Disabled  IntegratorVariant=Disabled  SatVariant=Disabled  AWVariant=Disabled  PCopyVariant=Disabled  TRVariant=Disabled  FdbkBlocksVariant=Forward  IdealPFdbkVariant=Disabled  SatFdbkVariant=Disabled  DerivativeFilterVariant=Disabled  NVariant=Disabled  NCopyVariant=Disabled_SignalSpec  FilterICVariant=Disabled  IntegratorICVariant=Disabled  ExternalResetVariant=Disabled  TRSumVariant=Passthrough  SumFdbkVariant=Disabled  SumVariant=Passthrough_P  TsampFilterVariant=InternalTs  TsampNgainVariant=Passthrough  TsampIntegralVariant=Disabled_SignalSpec  ExternalSaturationOutDataTypeStr=Inherit: Same as second input  DerivativeSourceVariant=Disabled  PreIntVariant=InternalPreInt
  Roll Rate controller : slpidlib/PID Controller  Controller=PD  Form=Parallel  TimeDomain=Continuous-time  UseExternalTs=off  SampleTime=-1  IntegratorMethod=Forward Euler  FilterMethod=Forward Euler  ControllerParametersSource=internal  P=0.213  I=8.92  UseKiTs=off  D=0.000599  UseExternalDerivativeSource=off  N=100  UseFilter=on  TunerSelectOption=Transfer Function Based (PID Tuner App)  InitialConditionSource=internal  InitialConditionForIntegrator=0  InitialConditionForFilter=0  DifferentiatorICPrevScaledInput=0  ExternalReset=none  TrackingMode=off  Kt=1  LimitOutput=off  SatLimitsSource=internal  UpperSaturationLimit=inf  LowerSaturationLimit=-inf  LinearizeAsGain=on  AntiWindupMode=none  Kb=1  LimitIntegrator=off  UpperIntegratorSaturationLimit=inf  LowerIntegratorSaturationLimit=-inf  POutMin=[]  POutMax=[]  IOutMin=[]  IOutMax=[]  DOutMin=[]  DOutMax=[]  NOutMin=[]  NOutMax=[]  SumOutMin=[]  SumOutMax=[]  SaturationOutMin=[]  SaturationOutMax=[]  PParamMin=[]  PParamMax=[]  IParamMin=[]  IParamMax=[]  DParamMin=[]  DParamMax=[]  NParamMin=[]  NParamMax=[]  KbParamMin=[]  KbParamMax=[]  KtParamMin=[]  KtParamMax=[]  KbOutMin=[]  KbOutMax=[]  KtOutMin=[]  KtOutMax=[]  IntegratorOutMin=[]  IntegratorOutMax=[]  FilterOutMin=[]  FilterOutMax=[]  SumI1OutMin=[]  SumI1OutMax=[]  SumI2OutMin=[]  SumI2OutMax=[]  SumI3OutMin=[]  SumI3OutMax=[]  SumI4OutMin=[]  SumI4OutMax=[]  SumDOutMin=[]  SumDOutMax=[]  DifferentiatorOutMin=[]  DifferentiatorOutMax=[]  FilterDiffOutCoefMin=[]  FilterDiffOutCoefMax=[]  ReciprocalOutMin=[]  ReciprocalOutMax=[]  SumDenOutMin=[]  SumDenOutMax=[]  SumNumOutMin=[]  SumNumOutMax=[]  DivideOutMin=[]  DivideOutMax=[]  UdiffTsProdOutMin=[]  UdiffTsProdOutMax=[]  NTsProdOutMin=[]  NTsProdOutMax=[]  UintegralTsProdOutMin=[]  UintegralTsProdOutMax=[]  UngainTsProdOutMin=[]  UngainTsProdOutMax=[]  ClampingZeroOutDataTypeStr=Inherit: Inherit via back propagation  ClampingZeroOutMin=[]  ClampingZeroOutMax=[]  FilterDenConstantOutDataTypeStr=Inherit: Inherit via back propagation  FilterDenConstantOutMin=[]  FilterDenConstantOutMax=[]  PCopyOutDataTypeStr=Inherit: Inherit via back propagation  PCopyOutMin=[]  PCopyOutMax=[]  NCopyOutDataTypeStr=Inherit: Inherit via back propagation  NCopyOutMin=[]  NCopyOutMax=[]  IntegratorContinuousStateAttributes=''  IntegratorStateMustResolveToSignalObject=off  IntegratorRTWStateStorageClass=Auto  FilterContinuousStateAttributes=''  FilterStateMustResolveToSignalObject=off  FilterRTWStateStorageClass=Auto  ParallelPVariant=InternalParameters  IdealPVariant=Disabled  IVariant=Disabled  DVariant=InternalParameters  IntegratorVariant=Disabled  SatVariant=Disabled  AWVariant=Disabled  PCopyVariant=Disabled  TRVariant=Disabled  FdbkBlocksVariant=Forward  IdealPFdbkVariant=Disabled  SatFdbkVariant=Disabled  DerivativeFilterVariant=ContFilter  NVariant=InternalParameters  NCopyVariant=Disabled  FilterICVariant=InternalICsFilter  IntegratorICVariant=Disabled  ExternalResetVariant=Disabled  TRSumVariant=Passthrough  SumFdbkVariant=Disabled  SumVariant=Sum_PD  TsampFilterVariant=InternalTs  TsampNgainVariant=Passthrough  TsampIntegralVariant=Disabled_SignalSpec  ExternalSaturationOutDataTypeStr=Inherit: Same as second input  DerivativeSourceVariant=ErrorSignal  PreIntVariant=InternalPreInt
  Roll Rate controller1 : slpidlib/PID Controller  Controller=P  Form=Parallel  TimeDomain=Continuous-time  UseExternalTs=off  SampleTime=-1  IntegratorMethod=Forward Euler  FilterMethod=Forward Euler  ControllerParametersSource=internal  P=0.0568  I=8.92  UseKiTs=off  D=0.0159  UseExternalDerivativeSource=off  N=50  UseFilter=on  TunerSelectOption=Transfer Function Based (PID Tuner App)  InitialConditionSource=internal  InitialConditionForIntegrator=0  InitialConditionForFilter=0  DifferentiatorICPrevScaledInput=0  ExternalReset=none  TrackingMode=off  Kt=1  LimitOutput=off  SatLimitsSource=internal  UpperSaturationLimit=inf  LowerSaturationLimit=-inf  LinearizeAsGain=on  AntiWindupMode=none  Kb=1  LimitIntegrator=off  UpperIntegratorSaturationLimit=inf  LowerIntegratorSaturationLimit=-inf  POutMin=[]  POutMax=[]  IOutMin=[]  IOutMax=[]  DOutMin=[]  DOutMax=[]  NOutMin=[]  NOutMax=[]  SumOutMin=[]  SumOutMax=[]  SaturationOutMin=[]  SaturationOutMax=[]  PParamMin=[]  PParamMax=[]  IParamMin=[]  IParamMax=[]  DParamMin=[]  DParamMax=[]  NParamMin=[]  NParamMax=[]  KbParamMin=[]  KbParamMax=[]  KtParamMin=[]  KtParamMax=[]  KbOutMin=[]  KbOutMax=[]  KtOutMin=[]  KtOutMax=[]  IntegratorOutMin=[]  IntegratorOutMax=[]  FilterOutMin=[]  FilterOutMax=[]  SumI1OutMin=[]  SumI1OutMax=[]  SumI2OutMin=[]  SumI2OutMax=[]  SumI3OutMin=[]  SumI3OutMax=[]  SumI4OutMin=[]  SumI4OutMax=[]  SumDOutMin=[]  SumDOutMax=[]  DifferentiatorOutMin=[]  DifferentiatorOutMax=[]  FilterDiffOutCoefMin=[]  FilterDiffOutCoefMax=[]  ReciprocalOutMin=[]  ReciprocalOutMax=[]  SumDenOutMin=[]  SumDenOutMax=[]  SumNumOutMin=[]  SumNumOutMax=[]  DivideOutMin=[]  DivideOutMax=[]  UdiffTsProdOutMin=[]  UdiffTsProdOutMax=[]  NTsProdOutMin=[]  NTsProdOutMax=[]  UintegralTsProdOutMin=[]  UintegralTsProdOutMax=[]  UngainTsProdOutMin=[]  UngainTsProdOutMax=[]  ClampingZeroOutDataTypeStr=Inherit: Inherit via back propagation  ClampingZeroOutMin=[]  ClampingZeroOutMax=[]  FilterDenConstantOutDataTypeStr=Inherit: Inherit via back propagation  FilterDenConstantOutMin=[]  FilterDenConstantOutMax=[]  PCopyOutDataTypeStr=Inherit: Inherit via back propagation  PCopyOutMin=[]  PCopyOutMax=[]  NCopyOutDataTypeStr=Inherit: Inherit via back propagation  NCopyOutMin=[]  NCopyOutMax=[]  IntegratorContinuousStateAttributes=''  IntegratorStateMustResolveToSignalObject=off  IntegratorRTWStateStorageClass=Auto  FilterContinuousStateAttributes=''  FilterStateMustResolveToSignalObject=off  FilterRTWStateStorageClass=Auto  ParallelPVariant=InternalParameters  IdealPVariant=Disabled  IVariant=Disabled  DVariant=Disabled  IntegratorVariant=Disabled  SatVariant=Disabled  AWVariant=Disabled  PCopyVariant=Disabled  TRVariant=Disabled  FdbkBlocksVariant=Forward  IdealPFdbkVariant=Disabled  SatFdbkVariant=Disabled  DerivativeFilterVariant=Disabled  NVariant=Disabled  NCopyVariant=Disabled_SignalSpec  FilterICVariant=Disabled  IntegratorICVariant=Disabled  ExternalResetVariant=Disabled  TRSumVariant=Passthrough  SumFdbkVariant=Disabled  SumVariant=Passthrough_P  TsampFilterVariant=InternalTs  TsampNgainVariant=Passthrough  TsampIntegralVariant=Disabled_SignalSpec  ExternalSaturationOutDataTypeStr=Inherit: Same as second input  DerivativeSourceVariant=Disabled  PreIntVariant=InternalPreInt
  Saturation1 : Saturate  UpperLimit=deg2rad(25)  LowerLimit=-deg2rad(25)
  Saturation2 : Saturate  UpperLimit=deg2rad(25)  LowerLimit=-deg2rad(25)
  Saturation4 : Saturate  UpperLimit=deg2rad(25)  LowerLimit=-deg2rad(25)
  Sum{1..6} (6 alike) : Sum  Inputs=|+-
  Yaw Angle controller : slpidlib/PID Controller  Controller=P  Form=Parallel  TimeDomain=Continuous-time  UseExternalTs=off  SampleTime=-1  IntegratorMethod=Forward Euler  FilterMethod=Forward Euler  ControllerParametersSource=internal  P=4.9  I=8.92  UseKiTs=off  D=0.101  UseExternalDerivativeSource=off  N=50  UseFilter=on  TunerSelectOption=Transfer Function Based (PID Tuner App)  InitialConditionSource=internal  InitialConditionForIntegrator=0  InitialConditionForFilter=0  DifferentiatorICPrevScaledInput=0  ExternalReset=none  TrackingMode=off  Kt=1  LimitOutput=off  SatLimitsSource=internal  UpperSaturationLimit=inf  LowerSaturationLimit=-inf  LinearizeAsGain=on  AntiWindupMode=none  Kb=1  LimitIntegrator=off  UpperIntegratorSaturationLimit=inf  LowerIntegratorSaturationLimit=-inf  POutMin=[]  POutMax=[]  IOutMin=[]  IOutMax=[]  DOutMin=[]  DOutMax=[]  NOutMin=[]  NOutMax=[]  SumOutMin=[]  SumOutMax=[]  SaturationOutMin=[]  SaturationOutMax=[]  PParamMin=[]  PParamMax=[]  IParamMin=[]  IParamMax=[]  DParamMin=[]  DParamMax=[]  NParamMin=[]  NParamMax=[]  KbParamMin=[]  KbParamMax=[]  KtParamMin=[]  KtParamMax=[]  KbOutMin=[]  KbOutMax=[]  KtOutMin=[]  KtOutMax=[]  IntegratorOutMin=[]  IntegratorOutMax=[]  FilterOutMin=[]  FilterOutMax=[]  SumI1OutMin=[]  SumI1OutMax=[]  SumI2OutMin=[]  SumI2OutMax=[]  SumI3OutMin=[]  SumI3OutMax=[]  SumI4OutMin=[]  SumI4OutMax=[]  SumDOutMin=[]  SumDOutMax=[]  DifferentiatorOutMin=[]  DifferentiatorOutMax=[]  FilterDiffOutCoefMin=[]  FilterDiffOutCoefMax=[]  ReciprocalOutMin=[]  ReciprocalOutMax=[]  SumDenOutMin=[]  SumDenOutMax=[]  SumNumOutMin=[]  SumNumOutMax=[]  DivideOutMin=[]  DivideOutMax=[]  UdiffTsProdOutMin=[]  UdiffTsProdOutMax=[]  NTsProdOutMin=[]  NTsProdOutMax=[]  UintegralTsProdOutMin=[]  UintegralTsProdOutMax=[]  UngainTsProdOutMin=[]  UngainTsProdOutMax=[]  ClampingZeroOutDataTypeStr=Inherit: Inherit via back propagation  ClampingZeroOutMin=[]  ClampingZeroOutMax=[]  FilterDenConstantOutDataTypeStr=Inherit: Inherit via back propagation  FilterDenConstantOutMin=[]  FilterDenConstantOutMax=[]  PCopyOutDataTypeStr=Inherit: Inherit via back propagation  PCopyOutMin=[]  PCopyOutMax=[]  NCopyOutDataTypeStr=Inherit: Inherit via back propagation  NCopyOutMin=[]  NCopyOutMax=[]  IntegratorContinuousStateAttributes=''  IntegratorStateMustResolveToSignalObject=off  IntegratorRTWStateStorageClass=Auto  FilterContinuousStateAttributes=''  FilterStateMustResolveToSignalObject=off  FilterRTWStateStorageClass=Auto  ParallelPVariant=InternalParameters  IdealPVariant=Disabled  IVariant=Disabled  DVariant=Disabled  IntegratorVariant=Disabled  SatVariant=Disabled  AWVariant=Disabled  PCopyVariant=Disabled  TRVariant=Disabled  FdbkBlocksVariant=Forward  IdealPFdbkVariant=Disabled  SatFdbkVariant=Disabled  DerivativeFilterVariant=Disabled  NVariant=Disabled  NCopyVariant=Disabled_SignalSpec  FilterICVariant=Disabled  IntegratorICVariant=Disabled  ExternalResetVariant=Disabled  TRSumVariant=Passthrough  SumFdbkVariant=Disabled  SumVariant=Passthrough_P  TsampFilterVariant=InternalTs  TsampNgainVariant=Passthrough  TsampIntegralVariant=Disabled_SignalSpec  ExternalSaturationOutDataTypeStr=Inherit: Same as second input  DerivativeSourceVariant=Disabled  PreIntVariant=InternalPreInt
  Yaw Rate controller : slpidlib/PID Controller  Controller=PD  Form=Parallel  TimeDomain=Continuous-time  UseExternalTs=off  SampleTime=-1  IntegratorMethod=Forward Euler  FilterMethod=Forward Euler  ControllerParametersSource=internal  P=6.66  I=8.92  UseKiTs=off  D=0.00933  UseExternalDerivativeSource=off  N=50  UseFilter=on  TunerSelectOption=Transfer Function Based (PID Tuner App)  InitialConditionSource=internal  InitialConditionForIntegrator=0  InitialConditionForFilter=0  DifferentiatorICPrevScaledInput=0  ExternalReset=none  TrackingMode=off  Kt=1  LimitOutput=off  SatLimitsSource=internal  UpperSaturationLimit=inf  LowerSaturationLimit=-inf  LinearizeAsGain=on  AntiWindupMode=none  Kb=1  LimitIntegrator=off  UpperIntegratorSaturationLimit=inf  LowerIntegratorSaturationLimit=-inf  POutMin=[]  POutMax=[]  IOutMin=[]  IOutMax=[]  DOutMin=[]  DOutMax=[]  NOutMin=[]  NOutMax=[]  SumOutMin=[]  SumOutMax=[]  SaturationOutMin=[]  SaturationOutMax=[]  PParamMin=[]  PParamMax=[]  IParamMin=[]  IParamMax=[]  DParamMin=[]  DParamMax=[]  NParamMin=[]  NParamMax=[]  KbParamMin=[]  KbParamMax=[]  KtParamMin=[]  KtParamMax=[]  KbOutMin=[]  KbOutMax=[]  KtOutMin=[]  KtOutMax=[]  IntegratorOutMin=[]  IntegratorOutMax=[]  FilterOutMin=[]  FilterOutMax=[]  SumI1OutMin=[]  SumI1OutMax=[]  SumI2OutMin=[]  SumI2OutMax=[]  SumI3OutMin=[]  SumI3OutMax=[]  SumI4OutMin=[]  SumI4OutMax=[]  SumDOutMin=[]  SumDOutMax=[]  DifferentiatorOutMin=[]  DifferentiatorOutMax=[]  FilterDiffOutCoefMin=[]  FilterDiffOutCoefMax=[]  ReciprocalOutMin=[]  ReciprocalOutMax=[]  SumDenOutMin=[]  SumDenOutMax=[]  SumNumOutMin=[]  SumNumOutMax=[]  DivideOutMin=[]  DivideOutMax=[]  UdiffTsProdOutMin=[]  UdiffTsProdOutMax=[]  NTsProdOutMin=[]  NTsProdOutMax=[]  UintegralTsProdOutMin=[]  UintegralTsProdOutMax=[]  UngainTsProdOutMin=[]  UngainTsProdOutMax=[]  ClampingZeroOutDataTypeStr=Inherit: Inherit via back propagation  ClampingZeroOutMin=[]  ClampingZeroOutMax=[]  FilterDenConstantOutDataTypeStr=Inherit: Inherit via back propagation  FilterDenConstantOutMin=[]  FilterDenConstantOutMax=[]  PCopyOutDataTypeStr=Inherit: Inherit via back propagation  PCopyOutMin=[]  PCopyOutMax=[]  NCopyOutDataTypeStr=Inherit: Inherit via back propagation  NCopyOutMin=[]  NCopyOutMax=[]  IntegratorContinuousStateAttributes=''  IntegratorStateMustResolveToSignalObject=off  IntegratorRTWStateStorageClass=Auto  FilterContinuousStateAttributes=''  FilterStateMustResolveToSignalObject=off  FilterRTWStateStorageClass=Auto  ParallelPVariant=InternalParameters  IdealPVariant=Disabled  IVariant=Disabled  DVariant=InternalParameters  IntegratorVariant=Disabled  SatVariant=Disabled  AWVariant=Disabled  PCopyVariant=Disabled  TRVariant=Disabled  FdbkBlocksVariant=Forward  IdealPFdbkVariant=Disabled  SatFdbkVariant=Disabled  DerivativeFilterVariant=ContFilter  NVariant=InternalParameters  NCopyVariant=Disabled  FilterICVariant=InternalICsFilter  IntegratorICVariant=Disabled  ExternalResetVariant=Disabled  TRSumVariant=Passthrough  SumFdbkVariant=Disabled  SumVariant=Sum_PD  TsampFilterVariant=InternalTs  TsampNgainVariant=Passthrough  TsampIntegralVariant=Disabled_SignalSpec  ExternalSaturationOutDataTypeStr=Inherit: Same as second input  DerivativeSourceVariant=ErrorSignal  PreIntVariant=InternalPreInt
  Roll Control Torque : Outport
  Pitch Control Torque : Outport  Port=2
  Yaw Control Torque : Outport  Port=3
  tag scope: mc_phi_desired=global, mc_psi_desired=global, mc_theta_desired=global
  wires:
  [theta_rad] -> Sum4/2
  Sum4/1 -> Pitch Angle controller/1
  Saturation4/1 -> Sum4/1
  Pitch Rate controller/1 -> Pitch Control Torque/1
  Sum1/1 -> Pitch Rate controller/1
  Pitch Angle controller/1 -> Sum1/1
  [q_rads] -> Sum1/2
  Theta_desired/1 -> [mc_theta_desired], Saturation4/1
  Phi_desired/1 -> [mc_phi_desired], Saturation1/1
  [phi_rad] -> Sum3/2
  Roll Rate controller/1 -> Roll Control Torque/1
  Saturation1/1 -> Sum3/1
  Sum3/1 -> Roll Angle controller/1
  [p_rads] -> Sum2/2
  Sum2/1 -> Roll Rate controller/1
  Roll Angle controller/1 -> Sum2/1
  Psi_desired/1 -> [mc_psi_desired], Saturation2/1
  [psi_rad] -> Sum6/2
  Yaw Rate controller/1 -> Yaw Control Torque/1
  Saturation2/1 -> Sum6/1
  Sum6/1 -> Yaw Angle controller/1
  [r_rads] -> Sum5/2
  Sum5/1 -> Yaw Rate controller/1
  Yaw Angle controller/1 -> Sum5/1

== system VTOL_quadplane/Autopilot ==
  Speed_desired : Inport
  Course Desired : Inport  Port=2
  Height Desired : Inport  Port=3
  Attitude Controller : Subsystem
  Beta_desired : Constant  Value=0
  Constant : Constant  Commented=on  Value=params  OutDataTypeStr=Bus: slBus1
  Constant1 : Constant  Commented=on  Value=0.707
  Constant2 : Constant  Commented=on  Value=deg2rad(15)
  Constant3 : Constant  Commented=on  Value=deg2rad(25)
  Constant4 : Constant  Commented=on  Value=deg2rad(10)
  From : From  Commented=on  GotoTag=TAS_mps  TagVisibility=global
  From1 : From  Commented=on  GotoTag=q_rads  TagVisibility=global
  From2 : From  Commented=on  GotoTag=theta_rad  TagVisibility=global
  Height Controller : Subsystem
  MATLAB Function : MATLAB Function  Commented=on  TreatAsAtomicUnit=on
  Product : Product
  Del_a : Outport
  Del_e : Outport  Port=2
  Del_r : Outport  Port=3
  Del_T : Outport  Port=4
  tag scope: del_T_controller=global, del_a_controller=global, del_e_controller=global, del_r_controller=global
  wires:
  Beta_desired/1 -> Attitude Controller/3(Beta_desired)  "Beta_desired"
  Course Desired/1 -> Height Controller/2(Course Desired)
  Attitude Controller/1(Del_a) -> Del_a/1, [del_a_controller]
  Height Controller/1(Del_T) -> Del_T/1, [del_T_controller]
  Attitude Controller/3(Del_r) -> Del_r/1, [del_r_controller]
  Height Controller/2(Phi_desired) -> Attitude Controller/1(Phi_desired)  "Phi_desired"
  Height Desired/1 -> Height Controller/3(Height Desired)
  Speed_desired/1 -> Height Controller/1(Speed_desired)
  Constant/1 -> MATLAB Function/5(params)
  From/1 -> MATLAB Function/4(Va)
  From1/1 -> MATLAB Function/3(q)
  From2/1 -> MATLAB Function/2(theta)
  Constant1/1 -> MATLAB Function/6(zeta_theta)
  Constant2/1 -> MATLAB Function/7(theta_e_max)
  Constant3/1 -> MATLAB Function/8(delta_e_max)
  Constant4/1 -> MATLAB Function/1(theta_c)
  Attitude Controller/2(Del_e) -> [del_e_controller], Del_e/1
  Height Controller/3(Thetha_desired) -> Product/1  "Theta_desired"
  [lambda] -> Product/2
  Product/1 -> Attitude Controller/2(Theta_desired)
